simulink model "MMCs_SingleCore"  (R2021b)
settings: Solver=FixedStepDiscrete  StartTime=0.0  StopTime=50  FixedStep=Ts  RelTol=1e-3  EnableMultiTasking=on
InitFcn:
  | MMCs_Parameters;
undefined symbols (not defined in the file): bias, Csm, DiscIntNeverNeededParam, Ki_cc, Ki_E1, Ki_E2, Ki_I, Ki_U, Kp_cc, Kp_E1, Kp_E2, Kp_I, Kp_U, Kr_cc, Kr_I, Kr_U, Nsm, Ts, Vdc, Vout, Vsm, w
libraries: raspberrypiCommlib x7, eeGeneralControl x6, slpidlib x6
settings Model: SimulationMode=external  Creator=s1941852  LastModifiedBy=s1941852
settings SolverCC: PositivePriorityOrder=on  AutoInsertRateTranBlk=on
settings OptimizationCC: EnhancedBackFolding=on  PassReuseOutputArgsAs=Individual arguments  ZeroExternalMemoryAtStartup=off  ZeroInternalMemoryAtStartup=off  MaxStackSize=64  OptimizeBlockOrder=speed  DifferentSizesBufferReuse=on  OptimizationCustomize=off  EfficientTunableParamExpr=on
settings DebuggingCC: ParameterTunabilityLossMsg=error
settings HardwareCC: ProdBitPerPointer=32  ProdBitPerSizeT=32  ProdBitPerPtrDiffT=32  ProdLargestAtomicInteger=Long  ProdLargestAtomicFloat=Double  ProdWordSize=32  ProdLongLongMode=on  ProdHWDeviceType=ARM Compatible->ARM Cortex
settings RTWCC: Description=Embedded Coder  SystemTargetFile=ert.tlc  HardwareBoard=Raspberry Pi  TLCOptions="-aInlineSetEventsForThisBaseRateFcn=TLC_FALSE -aSuppressMultiTaskScheduler=TLC_FALSE  -aRateBasedStepFcn=0"  TemplateMakefile=ert_default_tmf  Toolchain=GNU GCC Embedded Linux  BuildConfiguration=Faster Runs
settings CodeAppCC: ForceParamTrailComments=on  IgnoreCustomStorageClasses=off  OperatorAnnotations=on  SimulinkDataObjDesc=on  SFDataObjDesc=on  InsertBlockDesc=on
settings ERTTargetCC: SupportContinuousTime=on  SupportVariableSizeSignals=on  ExtModeTransport=2  ExtModeStaticAlloc=on  ExtModeMexFile=ext_xcp  ExtModeIntrfLevel=Level2 - Open

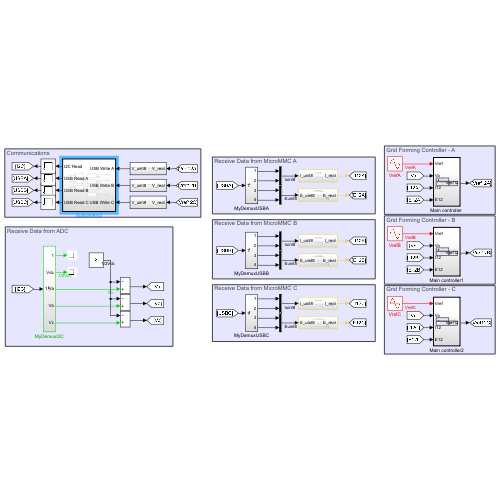
[thumbnail: Simulink's stored preview of the top-level diagram]
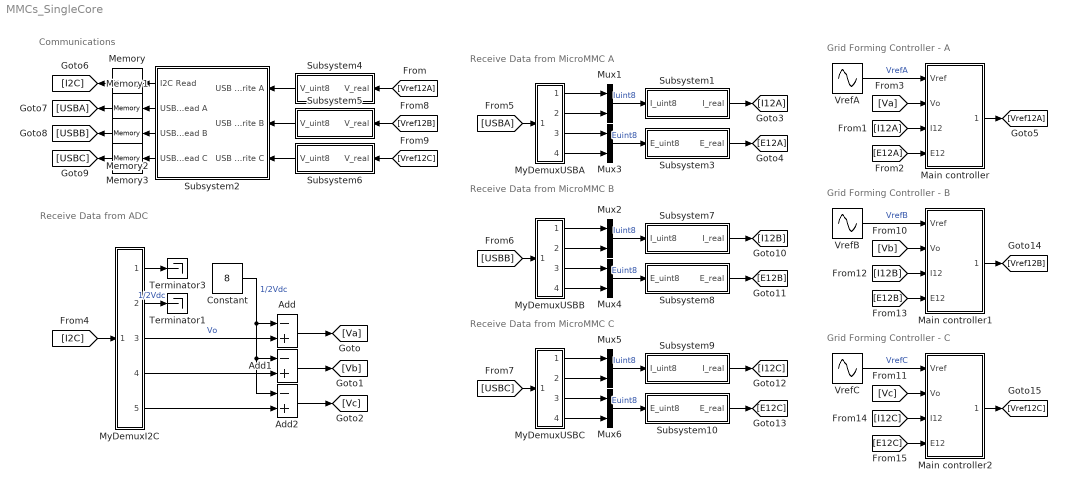
== system MMCs_SingleCore ==
  note: Communications
  note: Grid Forming Controller - A
  note: Receive Data from MicroMMC A
  note: Receive Data from ADC
  note: Grid Forming Controller - B
  note: Grid Forming Controller - C
  note: Receive Data from MicroMMC B
  note: Receive Data from MicroMMC C
  Add : Sum  Inputs=-+
  Add1 : Sum  Inputs=-+
  Add2 : Sum  Inputs=-+
  Constant : Constant  Value=8
  "Main controller " : Subsystem  TreatAsAtomicUnit=on  SystemSampleTime=Ts
  Main controller1 : Subsystem  TreatAsAtomicUnit=on  SystemSampleTime=Ts
  Main controller2 : Subsystem  TreatAsAtomicUnit=on  SystemSampleTime=Ts
  Memory{,1..3} (4 alike) : Memory
  Mux{1..6} (6 alike) : Mux  Inputs=2
  MyDemuxI2C : Subsystem
  MyDemuxUSBA : Subsystem
  MyDemuxUSBB : Subsystem
  MyDemuxUSBC : Subsystem
  Subsystem1 : Subsystem
  Subsystem10 : Subsystem
  Subsystem2 : Subsystem  TreatAsAtomicUnit=on  SystemSampleTime=Ts
      settings: PortSchema="{\"entries\":[{\"content\":{\"sides\":[{\"content\":{\"connectorIds\":[\"Out1\",\"Out2\",\"Out3\",\"Out4\"]},\"type\":\"ConnectorPlacement.EquallySpacedRectSide\",\"uuid\":\"46029ead-0964-4ae9-b883-4a06573532e6\"},{\"content\":{\"connectorIds\":[\"In1\",\"In2\",\"In3\"],\"side\":\"RIGHT\"},\"type\":\"ConnectorPlacement.EquallySpacedRectSide\",\"uuid\":\"15f59cbf-3bfc-4c74-a2e0-6efc08c03cef\"},{\"content\":{\"connectorIds\":[],\"side\":\"TOP\"},\"type\":\"ConnectorPlacement.EquallySpacedRectSide\",\"uuid\":\"8f43b052-da8c-4b5e-b754-50c4f07df149\"}]},\"type\":\"ConnectorPlacement.EquallySpacedConnector\",\"uuid\":\"6541cb38-b92e-4f8c-a13a-509f214bb128\"}],\"packageUris\":[\"http://schema.mathworks.com/mf0/Connector/R2020b\"],\"version\":\"1.0\"}"
  Subsystem3 : Subsystem
  Subsystem4 : Subsystem
  Subsystem5 : Subsystem
  Subsystem6 : Subsystem
  Subsystem7 : Subsystem
  Subsystem8 : Subsystem
  Subsystem9 : Subsystem
  Terminator1 : Terminator
  Terminator3 : Terminator
  VrefA : Sin  Amplitude=Vout  Bias=bias  Frequency=w  SampleTime=0
  VrefB : Sin  Amplitude=Vout  Bias=bias  Frequency=w  Phase=2/3*pi  SampleTime=0
  VrefC : Sin  Amplitude=Vout  Bias=bias  Frequency=w  Phase=4/3*pi  SampleTime=0
  wires:
  MyDemuxUSBA/2(Out2) -> Mux1/2
  MyDemuxUSBA/1(Out1) -> Mux1/1
  Mux1/1 -> Subsystem1/1(I_uint8)  "Iuint8"
  MyDemuxUSBA/4(Out4) -> Mux3/2
  MyDemuxUSBA/3(Out3) -> Mux3/1
  [I2C] -> MyDemuxI2C/1(In1)
  VrefA/1 -> "Main controller "/1(Vref)  "VrefA"
  [USBA] -> MyDemuxUSBA/1(In1)
  MyDemuxI2C/3(Va) -> Add/2  "Vo"
  Subsystem4/1(V_uint8) -> Subsystem2/1(USB Write A)
  MyDemuxI2C/1(Out1) -> Terminator3/1
  MyDemuxI2C/4(Vb) -> Add1/2
  MyDemuxI2C/5(Vc) -> Add2/2
  Mux3/1 -> Subsystem3/1(E_uint8)  "Euint8"
  Constant/1 -> Add/1, Add2/1, Add1/1  "1/2Vdc"
  [Vref12A] -> Subsystem4/1(V_real)
  Add/1 -> [Va]
  Add1/1 -> [Vb]
  Add2/1 -> [Vc]
  Subsystem5/1(V_uint8) -> Subsystem2/2(USB Write B)
  Subsystem6/1(V_uint8) -> Subsystem2/3(USB Write C)
  Subsystem1/1(I_real) -> [I12A]
  Subsystem3/1(E_real) -> [E12A]
  "Main controller "/1(Vref12) -> [Vref12A]
  [I12A] -> "Main controller "/3(I12)
  [E12A] -> "Main controller "/4(E12)
  [Va] -> "Main controller "/2(Vo)
  [Vb] -> Main controller1/2(Vo)
  [E12B] -> Main controller1/4(E12)
  [I12B] -> Main controller1/3(I12)
  Main controller1/1(Vref12) -> [Vref12B]
  VrefB/1 -> Main controller1/1(Vref)  "VrefB"
  VrefC/1 -> Main controller2/1(Vref)  "VrefC"
  Main controller2/1(Vref12) -> [Vref12C]
  [I12C] -> Main controller2/3(I12)
  [E12C] -> Main controller2/4(E12)
  [Vc] -> Main controller2/2(Vo)
  Subsystem8/1(E_real) -> [E12B]
  Subsystem7/1(I_real) -> [I12B]
  Mux4/1 -> Subsystem8/1(E_uint8)  "Euint8"
  MyDemuxUSBB/3(Out3) -> Mux4/1
  MyDemuxUSBB/4(Out4) -> Mux4/2
  Mux2/1 -> Subsystem7/1(I_uint8)  "Iuint8"
  MyDemuxUSBB/1(Out1) -> Mux2/1
  MyDemuxUSBB/2(Out2) -> Mux2/2
  MyDemuxUSBC/2(Out2) -> Mux5/2
  MyDemuxUSBC/1(Out1) -> Mux5/1
  Mux5/1 -> Subsystem9/1(I_uint8)  "Iuint8"
  MyDemuxUSBC/4(Out4) -> Mux6/2
  MyDemuxUSBC/3(Out3) -> Mux6/1
  Mux6/1 -> Subsystem10/1(E_uint8)  "Euint8"
  Subsystem9/1(I_real) -> [I12C]
  Subsystem10/1(E_real) -> [E12C]
  [USBB] -> MyDemuxUSBB/1(In1)
  [USBC] -> MyDemuxUSBC/1(In1)
  [Vref12B] -> Subsystem5/1(V_real)
  [Vref12C] -> Subsystem6/1(V_real)
  MyDemuxI2C/2(Vdc) -> Terminator1/1  "1/2Vdc"
  Memory/1 -> [I2C]
  Subsystem2/1(I2C Read) -> Memory/1
  Memory1/1 -> [USBA]
  Subsystem2/2(USB Read A) -> Memory1/1
  Memory2/1 -> [USBB]
  Subsystem2/3(USB Read B) -> Memory2/1
  Memory3/1 -> [USBC]
  Subsystem2/4(USB Read C) -> Memory3/1

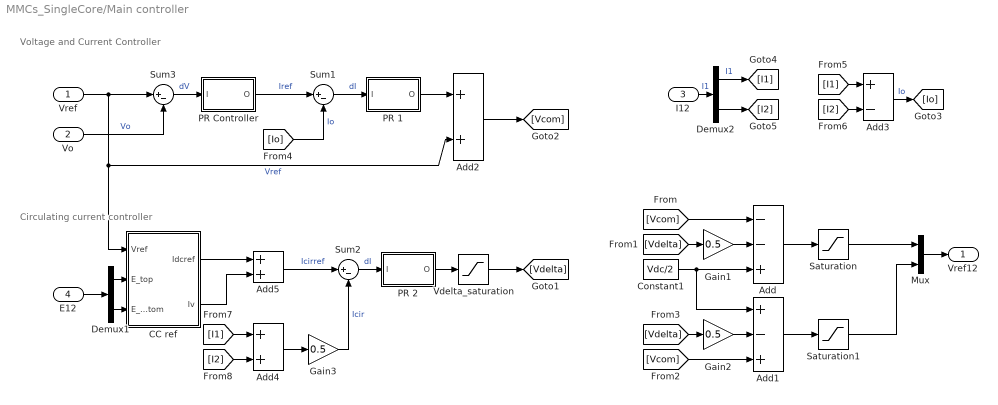
== system MMCs_SingleCore/Main controller  ==
  note: Voltage and Current Controller
  note: Circulating current controller
  Vref : Inport
  Vo : Inport  Port=2
  I12 : Inport  Port=3
  E12 : Inport  Port=4
  Add : Sum  Inputs=--+
  Add1 : Sum  Inputs=+-+
  Add2 : Sum
  Add3 : Sum  Inputs=+-
  Add4 : Sum
  Add5 : Sum
  CC ref : Subsystem
  Constant1 : Constant  Value=Vdc/2
  Demux1 : Demux  Outputs=2
  Demux2 : Demux  Outputs=2
  Gain1 : Gain  Gain=0.5
  Gain2 : Gain  Gain=0.5
  Gain3 : Gain  Gain=0.5
  Mux : Mux  Inputs=2
  PR 1 : Subsystem
  PR 2 : Subsystem
  PR Controller : Subsystem
  Saturation : Saturate  UpperLimit=16  LowerLimit=0
  Saturation1 : Saturate  UpperLimit=16  LowerLimit=0
  Sum1 : Sum  Inputs=|+-
  Sum2 : Sum  Inputs=|+-
  Sum3 : Sum  Inputs=|+-
  Vdelta_saturation : Saturate  UpperLimit=10  LowerLimit=-10
  Vref12 : Outport
  wires:
  Vref/1 -> Sum3/1, Add2/2, CC ref/1(Vref)  "Vref"
  Vo/1 -> Sum3/2  "Vo"
  Sum3/1 -> PR Controller/1(I)  "dV"
  PR Controller/1(O) -> Sum1/1  "Iref"
  [Io] -> Sum1/2  "Io"
  Sum1/1 -> PR 1/1(I)  "dI"
  [Vcom] -> Add/1
  Gain1/1 -> Add/2
  [Vdelta] -> Gain1/1
  [Vcom] -> Add1/3
  [Vdelta] -> Gain2/1
  Gain2/1 -> Add1/2
  Add2/1 -> [Vcom]
  Demux2/2 -> [I2]
  Add3/1 -> [Io]  "Io"
  Sum2/1 -> PR 2/1(I)  "dI"
  [I2] -> Add3/2
  [I1] -> Add3/1
  [I2] -> Add4/2
  Add4/1 -> Gain3/1
  [I1] -> Add4/1
  Add/1 -> Saturation/1
  Add1/1 -> Saturation1/1
  Vdelta_saturation/1 -> [Vdelta]
  Saturation/1 -> Mux/1
  Saturation1/1 -> Mux/2
  Demux2/1 -> [I1]  "I1"
  Constant1/1 -> Add1/1, Add/3
  Demux1/1 -> CC ref/2(E_top)
  Demux1/2 -> CC ref/3(E_bottom)
  Gain3/1 -> Sum2/2  "Icir"
  Add5/1 -> Sum2/1  "Icirref"
  CC ref/1(Idcref) -> Add5/1
  CC ref/2(Iv) -> Add5/2
  PR 1/1(O) -> Add2/1
  PR 2/1(O) -> Vdelta_saturation/1
  E12/1 -> Demux1/1
  I12/1 -> Demux2/1  "I1"
  Mux/1 -> Vref12/1

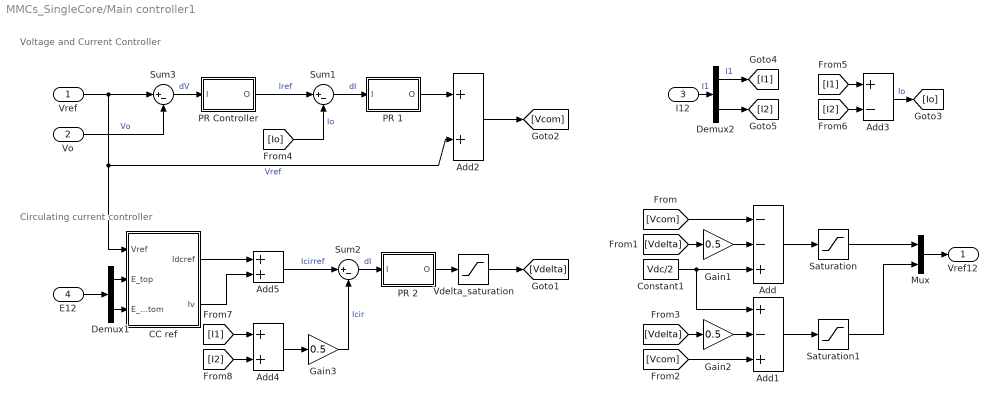
== system MMCs_SingleCore/Main controller1 ==
  note: Circulating current controller
  note: Voltage and Current Controller
  Vref : Inport
  Vo : Inport  Port=2
  I12 : Inport  Port=3
  E12 : Inport  Port=4
  Add : Sum  Inputs=--+
  Add1 : Sum  Inputs=+-+
  Add2 : Sum
  Add3 : Sum  Inputs=+-
  Add4 : Sum
  Add5 : Sum
  CC ref : Subsystem
  Constant1 : Constant  Value=Vdc/2
  Demux1 : Demux  Outputs=2
  Demux2 : Demux  Outputs=2
  Gain1 : Gain  Gain=0.5
  Gain2 : Gain  Gain=0.5
  Gain3 : Gain  Gain=0.5
  Mux : Mux  Inputs=2
  PR 1 : Subsystem
  PR 2 : Subsystem
  PR Controller : Subsystem
  Saturation : Saturate  UpperLimit=16  LowerLimit=0
  Saturation1 : Saturate  UpperLimit=16  LowerLimit=0
  Sum1 : Sum  Inputs=|+-
  Sum2 : Sum  Inputs=|+-
  Sum3 : Sum  Inputs=|+-
  Vdelta_saturation : Saturate  UpperLimit=10  LowerLimit=-10
  Vref12 : Outport
  wires:
  Mux/1 -> Vref12/1
  I12/1 -> Demux2/1  "I1"
  E12/1 -> Demux1/1
  PR 2/1(O) -> Vdelta_saturation/1
  PR 1/1(O) -> Add2/1
  CC ref/2(Iv) -> Add5/2
  CC ref/1(Idcref) -> Add5/1
  Add5/1 -> Sum2/1  "Icirref"
  Gain3/1 -> Sum2/2  "Icir"
  Demux1/2 -> CC ref/3(E_bottom)
  Demux1/1 -> CC ref/2(E_top)
  Constant1/1 -> Add/3, Add1/1
  Demux2/1 -> [I1]  "I1"
  Saturation1/1 -> Mux/2
  Saturation/1 -> Mux/1
  Vdelta_saturation/1 -> [Vdelta]
  Add1/1 -> Saturation1/1
  Add/1 -> Saturation/1
  [I1] -> Add4/1
  Add4/1 -> Gain3/1
  [I2] -> Add4/2
  [I1] -> Add3/1
  [I2] -> Add3/2
  Sum2/1 -> PR 2/1(I)  "dI"
  Add3/1 -> [Io]  "Io"
  Demux2/2 -> [I2]
  Add2/1 -> [Vcom]
  Gain2/1 -> Add1/2
  [Vdelta] -> Gain2/1
  [Vcom] -> Add1/3
  [Vdelta] -> Gain1/1
  Gain1/1 -> Add/2
  [Vcom] -> Add/1
  Sum1/1 -> PR 1/1(I)  "dI"
  [Io] -> Sum1/2  "Io"
  PR Controller/1(O) -> Sum1/1  "Iref"
  Sum3/1 -> PR Controller/1(I)  "dV"
  Vo/1 -> Sum3/2  "Vo"
  Vref/1 -> CC ref/1(Vref), Add2/2, Sum3/1  "Vref"

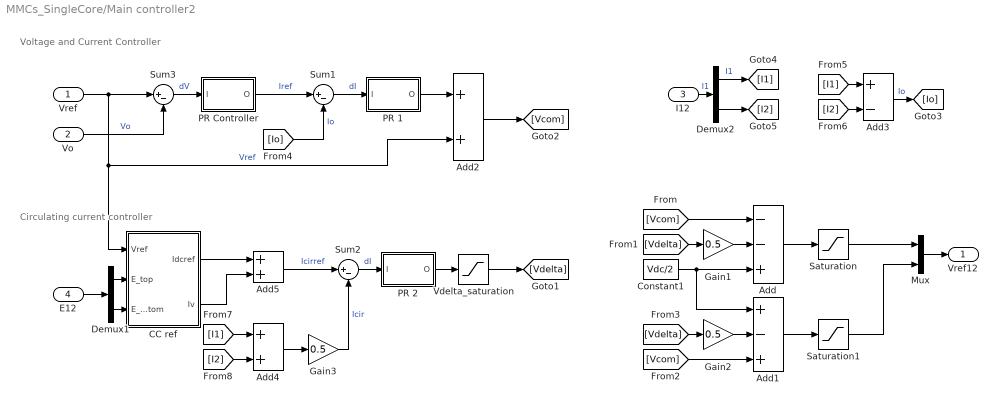
== system MMCs_SingleCore/Main controller2 ==
  note: Voltage and Current Controller
  note: Circulating current controller
  Vref : Inport
  Vo : Inport  Port=2
  I12 : Inport  Port=3
  E12 : Inport  Port=4
  Add : Sum  Inputs=--+
  Add1 : Sum  Inputs=+-+
  Add2 : Sum
  Add3 : Sum  Inputs=+-
  Add4 : Sum
  Add5 : Sum
  CC ref : Subsystem
  Constant1 : Constant  Value=Vdc/2
  Demux1 : Demux  Outputs=2
  Demux2 : Demux  Outputs=2
  Gain1 : Gain  Gain=0.5
  Gain2 : Gain  Gain=0.5
  Gain3 : Gain  Gain=0.5
  Mux : Mux  Inputs=2
  PR 1 : Subsystem
  PR 2 : Subsystem
  PR Controller : Subsystem
  Saturation : Saturate  UpperLimit=16  LowerLimit=0
  Saturation1 : Saturate  UpperLimit=16  LowerLimit=0
  Sum1 : Sum  Inputs=|+-
  Sum2 : Sum  Inputs=|+-
  Sum3 : Sum  Inputs=|+-
  Vdelta_saturation : Saturate  UpperLimit=10  LowerLimit=-10
  Vref12 : Outport
  wires:
  Vref/1 -> Sum3/1, Add2/2, CC ref/1(Vref)  "Vref"
  Vo/1 -> Sum3/2  "Vo"
  Sum3/1 -> PR Controller/1(I)  "dV"
  PR Controller/1(O) -> Sum1/1  "Iref"
  [Io] -> Sum1/2  "Io"
  Sum1/1 -> PR 1/1(I)  "dI"
  [Vcom] -> Add/1
  Gain1/1 -> Add/2
  [Vdelta] -> Gain1/1
  [Vcom] -> Add1/3
  [Vdelta] -> Gain2/1
  Gain2/1 -> Add1/2
  Add2/1 -> [Vcom]
  Demux2/2 -> [I2]
  Add3/1 -> [Io]  "Io"
  Sum2/1 -> PR 2/1(I)  "dI"
  [I2] -> Add3/2
  [I1] -> Add3/1
  [I2] -> Add4/2
  Add4/1 -> Gain3/1
  [I1] -> Add4/1
  Add/1 -> Saturation/1
  Add1/1 -> Saturation1/1
  Vdelta_saturation/1 -> [Vdelta]
  Saturation/1 -> Mux/1
  Saturation1/1 -> Mux/2
  Demux2/1 -> [I1]  "I1"
  Constant1/1 -> Add1/1, Add/3
  Demux1/1 -> CC ref/2(E_top)
  Demux1/2 -> CC ref/3(E_bottom)
  Gain3/1 -> Sum2/2  "Icir"
  Add5/1 -> Sum2/1  "Icirref"
  CC ref/1(Idcref) -> Add5/1
  CC ref/2(Iv) -> Add5/2
  PR 1/1(O) -> Add2/1
  PR 2/1(O) -> Vdelta_saturation/1
  E12/1 -> Demux1/1
  I12/1 -> Demux2/1  "I1"
  Mux/1 -> Vref12/1

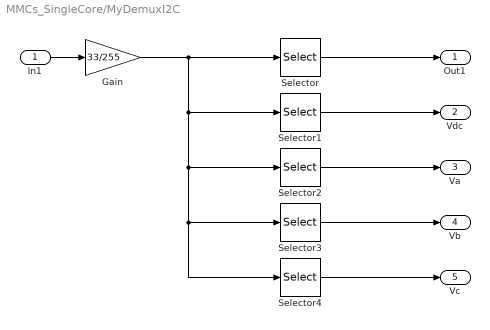
== system MMCs_SingleCore/MyDemuxI2C ==
  In1 : Inport
  Gain : Gain  Gain=33/255
  Selector : Selector  NumberOfDimensions=2  InputPortWidth=4  IndexOptions=Index vector (dialog),Index vector (dialog)  Indices=[1],1  OutputSizes=1,1
  Selector1 : Selector  NumberOfDimensions=2  InputPortWidth=4  IndexOptions=Index vector (dialog),Index vector (dialog)  Indices=[2],1  OutputSizes=1,1
  Selector2 : Selector  NumberOfDimensions=2  InputPortWidth=4  IndexOptions=Index vector (dialog),Index vector (dialog)  Indices=[3],1  OutputSizes=1,1
  Selector3 : Selector  NumberOfDimensions=2  InputPortWidth=4  IndexOptions=Index vector (dialog),Index vector (dialog)  Indices=[4],1  OutputSizes=1,1
  Selector4 : Selector  NumberOfDimensions=2  InputPortWidth=4  IndexOptions=Index vector (dialog),Index vector (dialog)  Indices=[5],1  OutputSizes=1,1
  Out1 : Outport
  Vdc : Outport  Port=2
  Va : Outport  Port=3
  Vb : Outport  Port=4
  Vc : Outport  Port=5
  wires:
  In1/1 -> Gain/1
  Selector1/1 -> Vdc/1
  Selector2/1 -> Va/1
  Selector3/1 -> Vb/1
  Selector/1 -> Out1/1
  Selector4/1 -> Vc/1
  Gain/1 -> Selector4/1, Selector3/1, Selector2/1, Selector1/1, Selector/1

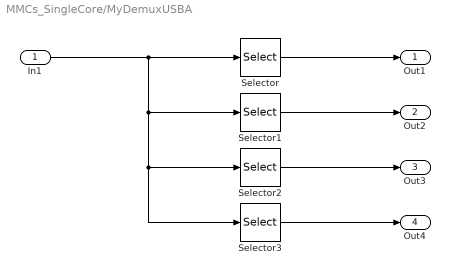
== system MMCs_SingleCore/MyDemuxUSBA ==
  In1 : Inport
  Selector : Selector  NumberOfDimensions=2  InputPortWidth=4  IndexOptions=Index vector (dialog),Index vector (dialog)  Indices=[1],1  OutputSizes=1,1
  Selector1 : Selector  NumberOfDimensions=2  InputPortWidth=4  IndexOptions=Index vector (dialog),Index vector (dialog)  Indices=[2],1  OutputSizes=1,1
  Selector2 : Selector  NumberOfDimensions=2  InputPortWidth=4  IndexOptions=Index vector (dialog),Index vector (dialog)  Indices=[3],1  OutputSizes=1,1
  Selector3 : Selector  NumberOfDimensions=2  InputPortWidth=4  IndexOptions=Index vector (dialog),Index vector (dialog)  Indices=[4],1  OutputSizes=1,1
  Out1 : Outport
  Out2 : Outport  Port=2
  Out3 : Outport  Port=3
  Out4 : Outport  Port=4
  wires:
  In1/1 -> Selector3/1, Selector2/1, Selector1/1, Selector/1
  Selector1/1 -> Out2/1
  Selector2/1 -> Out3/1
  Selector3/1 -> Out4/1
  Selector/1 -> Out1/1

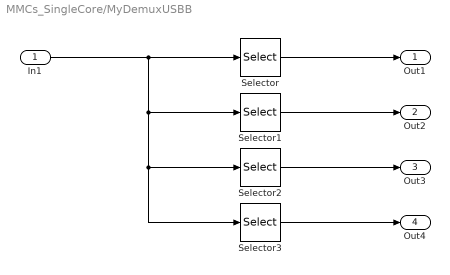
== system MMCs_SingleCore/MyDemuxUSBB ==
  In1 : Inport
  Selector : Selector  NumberOfDimensions=2  InputPortWidth=4  IndexOptions=Index vector (dialog),Index vector (dialog)  Indices=[1],1  OutputSizes=1,1
  Selector1 : Selector  NumberOfDimensions=2  InputPortWidth=4  IndexOptions=Index vector (dialog),Index vector (dialog)  Indices=[2],1  OutputSizes=1,1
  Selector2 : Selector  NumberOfDimensions=2  InputPortWidth=4  IndexOptions=Index vector (dialog),Index vector (dialog)  Indices=[3],1  OutputSizes=1,1
  Selector3 : Selector  NumberOfDimensions=2  InputPortWidth=4  IndexOptions=Index vector (dialog),Index vector (dialog)  Indices=[4],1  OutputSizes=1,1
  Out1 : Outport
  Out2 : Outport  Port=2
  Out3 : Outport  Port=3
  Out4 : Outport  Port=4
  wires:
  Selector/1 -> Out1/1
  Selector3/1 -> Out4/1
  Selector2/1 -> Out3/1
  Selector1/1 -> Out2/1
  In1/1 -> Selector/1, Selector1/1, Selector2/1, Selector3/1

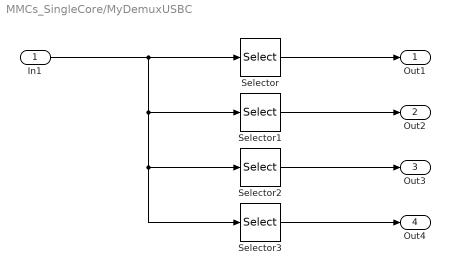
== system MMCs_SingleCore/MyDemuxUSBC ==
  In1 : Inport
  Selector : Selector  NumberOfDimensions=2  InputPortWidth=4  IndexOptions=Index vector (dialog),Index vector (dialog)  Indices=[1],1  OutputSizes=1,1
  Selector1 : Selector  NumberOfDimensions=2  InputPortWidth=4  IndexOptions=Index vector (dialog),Index vector (dialog)  Indices=[2],1  OutputSizes=1,1
  Selector2 : Selector  NumberOfDimensions=2  InputPortWidth=4  IndexOptions=Index vector (dialog),Index vector (dialog)  Indices=[3],1  OutputSizes=1,1
  Selector3 : Selector  NumberOfDimensions=2  InputPortWidth=4  IndexOptions=Index vector (dialog),Index vector (dialog)  Indices=[4],1  OutputSizes=1,1
  Out1 : Outport
  Out2 : Outport  Port=2
  Out3 : Outport  Port=3
  Out4 : Outport  Port=4
  wires:
  In1/1 -> Selector3/1, Selector2/1, Selector1/1, Selector/1
  Selector1/1 -> Out2/1
  Selector2/1 -> Out3/1
  Selector3/1 -> Out4/1
  Selector/1 -> Out1/1

== system MMCs_SingleCore/Subsystem1 ==
  note: (-3 to 3) --> (0 to 240)
      | (I_real + 3) * 40 = I_uint8
  I_uint8 : Inport
  Constant : Constant  Value=3  SampleTime=-1
  Convert to double : DataTypeConversion  OutDataTypeStr=double
  Gain : Gain  Gain=1/40
  Sum3 : Sum  Inputs=+-
  I_real : Outport
  wires:
  Gain/1 -> Sum3/1
  Convert to double/1 -> Gain/1
  Constant/1 -> Sum3/2
  I_uint8/1 -> Convert to double/1
  Sum3/1 -> I_real/1

== system MMCs_SingleCore/Subsystem10 ==
  note: (0 to 2.4) --> (0 to 120)
      | E_real * 50 = E_uint8
      | 4 * 1/2 * 3 * 6.8e-3 * 5^2 = 1.02 (51 in uint8)
  E_uint8 : Inport
  Convert to double : DataTypeConversion  OutDataTypeStr=double
  Gain : Gain  Gain=1/50
  Scope : Scope  NumInputPorts=3
  E_real : Outport
  wires:
  Gain/1 -> Scope/3, E_real/1
  E_uint8/1 -> Scope/1, Convert to double/1
  Convert to double/1 -> Scope/2, Gain/1

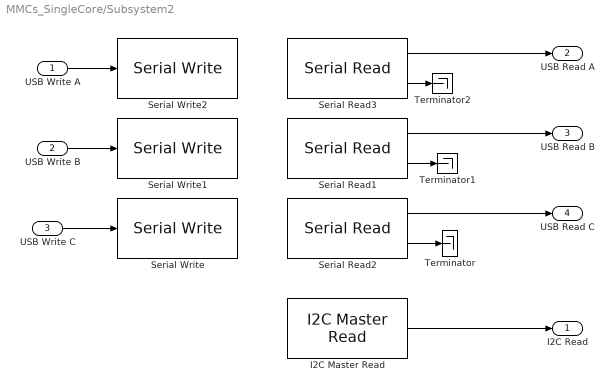
== system MMCs_SingleCore/Subsystem2 ==
  USB Write A : Inport
  USB Write B : Inport  Port=2
  USB Write C : Inport  Port=3
  I2C Master Read : raspberrypiCommlib/I2C Master Read  Priority=1  BoardProperty=Pi 4 Model B  Mode=Master  SlaveAddress=hex2dec('20')  SlaveByteOrder=BigEndian  Direction=Receiver  RegisterAddressMode=off  RegisterAddress=0b00000000  SlaveDataType=uint8  DataLength=5  NoAck=off  RepeatedStart=off  OutputStatus=off  SampleTime=-1
      settings: SourceProductBaseCode=RASPPI
  Serial Read1 : raspberrypiCommlib/Serial Read  Priority=5  board=Pi 4 Model B  SCIModule_=/dev/ttyACM1  Baudrate_=230400  Parity=None  StopBits_=1  HardwareFlowControl=None  ByteOrder=LittleEndian  DataLength=4  DataType=uint8  OutputStatus=on  SampleTime=-1  blockPlatform=RaspberryPi
      settings: SourceProductBaseCode=RASPPI
  Serial Read2 : raspberrypiCommlib/Serial Read  Priority=7  board=Pi 4 Model B  SCIModule_=/dev/ttyACM2  Baudrate_=230400  Parity=None  StopBits_=1  HardwareFlowControl=None  ByteOrder=LittleEndian  DataLength=4  DataType=uint8  OutputStatus=on  SampleTime=-1  blockPlatform=RaspberryPi
      settings: SourceProductBaseCode=RASPPI
  Serial Read3 : raspberrypiCommlib/Serial Read  Priority=3  board=Pi 4 Model B  SCIModule_=/dev/ttyACM0  Baudrate_=230400  Parity=None  StopBits_=1  HardwareFlowControl=None  ByteOrder=LittleEndian  DataLength=4  DataType=uint8  OutputStatus=on  SampleTime=-1  blockPlatform=RaspberryPi
      settings: SourceProductBaseCode=RASPPI
  Serial Write : raspberrypiCommlib/Serial Write  Priority=6  board=Pi 4 Model B  SCIModule_=/dev/ttyACM2  Baudrate_=230400  Parity=None  StopBits_=1  HardwareFlowControl=None  ByteOrder=LittleEndian  OutputStatus=off  blockPlatform=RaspberryPi
      settings: SourceProductBaseCode=RASPPI
  Serial Write1 : raspberrypiCommlib/Serial Write  Priority=4  board=Pi 4 Model B  SCIModule_=/dev/ttyACM1  Baudrate_=230400  Parity=None  StopBits_=1  HardwareFlowControl=None  ByteOrder=LittleEndian  OutputStatus=off  blockPlatform=RaspberryPi
      settings: SourceProductBaseCode=RASPPI
  Serial Write2 : raspberrypiCommlib/Serial Write  Priority=2  board=Pi 4 Model B  SCIModule_=/dev/ttyACM0  Baudrate_=230400  Parity=None  StopBits_=1  HardwareFlowControl=None  ByteOrder=LittleEndian  OutputStatus=off  blockPlatform=RaspberryPi
      settings: SourceProductBaseCode=RASPPI
  Terminator : Terminator
  Terminator1 : Terminator
  Terminator2 : Terminator
  I2C Read : Outport
  USB Read A : Outport  Port=2
  USB Read B : Outport  Port=3
  USB Read C : Outport  Port=4
  wires:
  I2C Master Read/1 -> I2C Read/1
  Serial Read2/2 -> Terminator/1
  Serial Read1/2 -> Terminator1/1
  Serial Read3/2 -> Terminator2/1
  USB Write A/1 -> Serial Write2/1
  Serial Read2/1 -> USB Read C/1
  USB Write B/1 -> Serial Write1/1
  Serial Read1/1 -> USB Read B/1
  USB Write C/1 -> Serial Write/1
  Serial Read3/1 -> USB Read A/1

== system MMCs_SingleCore/Subsystem3 ==
  note: (0 to 2.4) --> (0 to 120)
      | E_real * 50 = E_uint8
      | 4 * 1/2 * 3 * 6.8e-3 * 5^2 = 1.02 (51 in uint8)
  E_uint8 : Inport
  Convert to double : DataTypeConversion  OutDataTypeStr=double
  Gain : Gain  Gain=1/50
  Scope : Scope  NumInputPorts=3
  E_real : Outport
  wires:
  Gain/1 -> Scope/3, E_real/1
  E_uint8/1 -> Scope/1, Convert to double/1
  Convert to double/1 -> Scope/2, Gain/1

== system MMCs_SingleCore/Subsystem4 ==
  V_real : Inport
  Add : Sum
  Constant3 : Constant  Value=20
  Convert to logical1 : DataTypeConversion  OutDataTypeStr=uint8
  Gain : Gain  Gain=240/40
  Saturation1 : Saturate  UpperLimit=2^8-1  LowerLimit=0
  V_uint8 : Outport
  wires:
  Constant3/1 -> Add/2
  Convert to logical1/1 -> V_uint8/1
  Saturation1/1 -> Convert to logical1/1
  V_real/1 -> Add/1
  Add/1 -> Gain/1
  Gain/1 -> Saturation1/1

== system MMCs_SingleCore/Subsystem5 ==
  V_real : Inport
  Add : Sum
  Constant3 : Constant  Value=20
  Convert to logical1 : DataTypeConversion  OutDataTypeStr=uint8
  Gain : Gain  Gain=240/40
  Saturation1 : Saturate  UpperLimit=2^8-1  LowerLimit=0
  V_uint8 : Outport
  wires:
  Gain/1 -> Saturation1/1
  Add/1 -> Gain/1
  V_real/1 -> Add/1
  Saturation1/1 -> Convert to logical1/1
  Convert to logical1/1 -> V_uint8/1
  Constant3/1 -> Add/2

== system MMCs_SingleCore/Subsystem6 ==
  V_real : Inport
  Add : Sum
  Constant3 : Constant  Value=20
  Convert to logical1 : DataTypeConversion  OutDataTypeStr=uint8
  Gain : Gain  Gain=240/40
  Saturation1 : Saturate  UpperLimit=2^8-1  LowerLimit=0
  V_uint8 : Outport
  wires:
  Constant3/1 -> Add/2
  Convert to logical1/1 -> V_uint8/1
  Saturation1/1 -> Convert to logical1/1
  V_real/1 -> Add/1
  Add/1 -> Gain/1
  Gain/1 -> Saturation1/1

== system MMCs_SingleCore/Subsystem7 ==
  note: (-3 to 3) --> (0 to 240)
      | (I_real + 3) * 40 = I_uint8
  I_uint8 : Inport
  Constant : Constant  Value=3  SampleTime=-1
  Convert to double : DataTypeConversion  OutDataTypeStr=double
  Gain : Gain  Gain=1/40
  Sum3 : Sum  Inputs=+-
  I_real : Outport
  wires:
  Sum3/1 -> I_real/1
  I_uint8/1 -> Convert to double/1
  Constant/1 -> Sum3/2
  Convert to double/1 -> Gain/1
  Gain/1 -> Sum3/1

== system MMCs_SingleCore/Subsystem8 ==
  note: (0 to 2.4) --> (0 to 120)
      | E_real * 50 = E_uint8
      | 4 * 1/2 * 3 * 6.8e-3 * 5^2 = 1.02 (51 in uint8)
  E_uint8 : Inport
  Convert to double : DataTypeConversion  OutDataTypeStr=double
  Gain : Gain  Gain=1/50
  Scope : Scope  NumInputPorts=3
  E_real : Outport
  wires:
  Convert to double/1 -> Gain/1, Scope/2
  E_uint8/1 -> Convert to double/1, Scope/1
  Gain/1 -> E_real/1, Scope/3

== system MMCs_SingleCore/Subsystem9 ==
  note: (-3 to 3) --> (0 to 240)
      | (I_real + 3) * 40 = I_uint8
  I_uint8 : Inport
  Constant : Constant  Value=3  SampleTime=-1
  Convert to double : DataTypeConversion  OutDataTypeStr=double
  Gain : Gain  Gain=1/40
  Sum3 : Sum  Inputs=+-
  I_real : Outport
  wires:
  Gain/1 -> Sum3/1
  Convert to double/1 -> Gain/1
  Constant/1 -> Sum3/2
  I_uint8/1 -> Convert to double/1
  Sum3/1 -> I_real/1

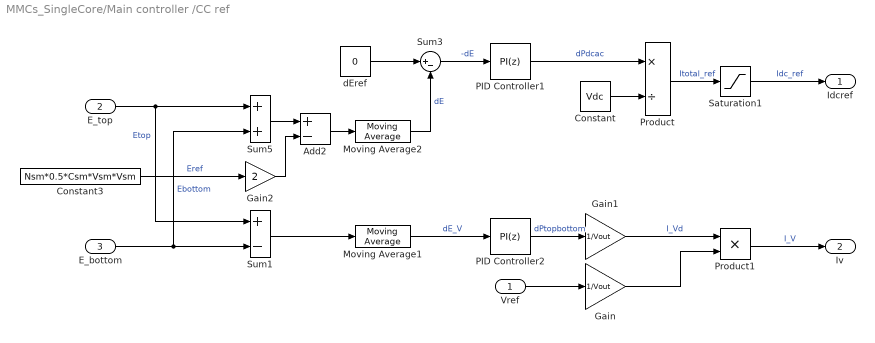
== system MMCs_SingleCore/Main controller /CC ref ==
  Vref : Inport
  E_top : Inport  Port=2
  E_bottom : Inport  Port=3
  Add2 : Sum  Inputs=+-
  Constant : Constant  Value=Vdc
  Constant3 : Constant  Value=Nsm*0.5*Csm*Vsm*Vsm
  Gain : Gain  Gain=1/Vout
  Gain1 : Gain  Gain=1/Vout
  Gain2 : Gain  Gain=2
  Moving Average1 : eeGeneralControl/Moving Average  VariantControl=Variant1  LabelModeActiveChoice=Discrete  f=5  x0=0  BufferSize=8192  Ts=Ts
      settings: SourceProductBaseCode=PS
  Moving Average2 : eeGeneralControl/Moving Average  VariantControl=Variant1  LabelModeActiveChoice=Discrete  f=5  x0=0  BufferSize=8192  Ts=Ts
      settings: SourceProductBaseCode=PS
  PID Controller1 : slpidlib/PID Controller  Controller=PI  Form=Parallel  TimeDomain=Discrete-time  UseExternalTs=off  SampleTime=-1  IntegratorMethod=Forward Euler  FilterMethod=Forward Euler  ControllerParametersSource=internal  P=Kp_E1  I=Ki_E1  D=0  UseFilter=on  N=100  TunerSelectOption=Transfer Function Based (PID Tuner App)  InitialConditionSource=internal  InitialConditionForIntegrator=0  InitialConditionForFilter=0  DifferentiatorICPrevScaledInput=0  ExternalReset=none  TrackingMode=off  Kt=1  LimitOutput=off  SatLimitsSource=internal  UpperSaturationLimit=inf  LowerSaturationLimit=-inf  LinearizeAsGain=on  AntiWindupMode=none  Kb=1  POutMin=[]  POutMax=[]  IOutMin=[]  IOutMax=[]  DOutMin=[]  DOutMax=[]  NOutMin=[]  NOutMax=[]  SumOutMin=[]  SumOutMax=[]  SaturationOutMin=[]  SaturationOutMax=[]  PParamMin=[]  PParamMax=[]  IParamMin=[]  IParamMax=[]  DParamMin=[]  DParamMax=[]  NParamMin=[]  NParamMax=[]  KbParamMin=[]  KbParamMax=[]  KtParamMin=[]  KtParamMax=[]  KbOutMin=[]  KbOutMax=[]  KtOutMin=[]  KtOutMax=[]  IntegratorOutMin=[]  IntegratorOutMax=[]  FilterOutMin=[]  FilterOutMax=[]  SumI1OutMin=[]  SumI1OutMax=[]  SumI2OutMin=[]  SumI2OutMax=[]  SumI3OutMin=[]  SumI3OutMax=[]  SumI4OutMin=[]  SumI4OutMax=[]  SumDOutMin=[]  SumDOutMax=[]  DifferentiatorOutMin=[]  DifferentiatorOutMax=[]  FilterDiffOutCoefMin=[]  FilterDiffOutCoefMax=[]  ReciprocalOutMin=[]  ReciprocalOutMax=[]  SumDenOutMin=[]  SumDenOutMax=[]  SumNumOutMin=[]  SumNumOutMax=[]  DivideOutMin=[]  DivideOutMax=[]  UdiffTsProdOutMin=[]  UdiffTsProdOutMax=[]  NTsProdOutMin=[]  NTsProdOutMax=[]  UintegralTsProdOutMin=[]  UintegralTsProdOutMax=[]  UngainTsProdOutMin=[]  UngainTsProdOutMax=[]  IntegratorContinuousStateAttributes=''  IntegratorStateMustResolveToSignalObject=off  IntegratorRTWStateStorageClass=Auto  FilterContinuousStateAttributes=''  FilterStateMustResolveToSignalObject=off  FilterRTWStateStorageClass=Auto  ParallelPVariant=InternalParameters  IdealPVariant=Disabled  IVariant=InternalParameters  DVariant=Disabled  IntegratorVariant=Discrete  SatVariant=Disabled  AWVariant=Passthrough  PCopyVariant=Disabled  TRVariant=Disabled  FdbkBlocksVariant=Forward  IdealPFdbkVariant=Disabled  SatFdbkVariant=Disabled  DerivativeFilterVariant=Disabled  NVariant=Disabled  NCopyVariant=Disabled_SignalSpec  FilterICVariant=Disabled  IntegratorICVariant=InternalICs  ExternalResetVariant=Disabled  TRSumVariant=Passthrough  SumFdbkVariant=Disabled  SumVariant=Sum_PI  TsampFilterVariant=InternalTs  TsampNgainVariant=Passthrough  TsampIntegralVariant=Passthrough  ExternalSaturationOutDataTypeStr=Inherit: Same as second input
  PID Controller2 : slpidlib/PID Controller  Controller=PI  Form=Parallel  TimeDomain=Discrete-time  UseExternalTs=off  SampleTime=-1  IntegratorMethod=Forward Euler  FilterMethod=Forward Euler  ControllerParametersSource=internal  P=Kp_E2  I=Ki_E2  D=0  UseFilter=on  N=100  TunerSelectOption=Transfer Function Based (PID Tuner App)  InitialConditionSource=internal  InitialConditionForIntegrator=0  InitialConditionForFilter=0  DifferentiatorICPrevScaledInput=0  ExternalReset=none  TrackingMode=off  Kt=1  LimitOutput=off  SatLimitsSource=internal  UpperSaturationLimit=inf  LowerSaturationLimit=-inf  LinearizeAsGain=on  AntiWindupMode=none  Kb=1  POutMin=[]  POutMax=[]  IOutMin=[]  IOutMax=[]  DOutMin=[]  DOutMax=[]  NOutMin=[]  NOutMax=[]  SumOutMin=[]  SumOutMax=[]  SaturationOutMin=[]  SaturationOutMax=[]  PParamMin=[]  PParamMax=[]  IParamMin=[]  IParamMax=[]  DParamMin=[]  DParamMax=[]  NParamMin=[]  NParamMax=[]  KbParamMin=[]  KbParamMax=[]  KtParamMin=[]  KtParamMax=[]  KbOutMin=[]  KbOutMax=[]  KtOutMin=[]  KtOutMax=[]  IntegratorOutMin=[]  IntegratorOutMax=[]  FilterOutMin=[]  FilterOutMax=[]  SumI1OutMin=[]  SumI1OutMax=[]  SumI2OutMin=[]  SumI2OutMax=[]  SumI3OutMin=[]  SumI3OutMax=[]  SumI4OutMin=[]  SumI4OutMax=[]  SumDOutMin=[]  SumDOutMax=[]  DifferentiatorOutMin=[]  DifferentiatorOutMax=[]  FilterDiffOutCoefMin=[]  FilterDiffOutCoefMax=[]  ReciprocalOutMin=[]  ReciprocalOutMax=[]  SumDenOutMin=[]  SumDenOutMax=[]  SumNumOutMin=[]  SumNumOutMax=[]  DivideOutMin=[]  DivideOutMax=[]  UdiffTsProdOutMin=[]  UdiffTsProdOutMax=[]  NTsProdOutMin=[]  NTsProdOutMax=[]  UintegralTsProdOutMin=[]  UintegralTsProdOutMax=[]  UngainTsProdOutMin=[]  UngainTsProdOutMax=[]  IntegratorContinuousStateAttributes=''  IntegratorStateMustResolveToSignalObject=off  IntegratorRTWStateStorageClass=Auto  FilterContinuousStateAttributes=''  FilterStateMustResolveToSignalObject=off  FilterRTWStateStorageClass=Auto  ParallelPVariant=InternalParameters  IdealPVariant=Disabled  IVariant=InternalParameters  DVariant=Disabled  IntegratorVariant=Discrete  SatVariant=Disabled  AWVariant=Passthrough  PCopyVariant=Disabled  TRVariant=Disabled  FdbkBlocksVariant=Forward  IdealPFdbkVariant=Disabled  SatFdbkVariant=Disabled  DerivativeFilterVariant=Disabled  NVariant=Disabled  NCopyVariant=Disabled_SignalSpec  FilterICVariant=Disabled  IntegratorICVariant=InternalICs  ExternalResetVariant=Disabled  TRSumVariant=Passthrough  SumFdbkVariant=Disabled  SumVariant=Sum_PI  TsampFilterVariant=InternalTs  TsampNgainVariant=Passthrough  TsampIntegralVariant=Passthrough  ExternalSaturationOutDataTypeStr=Inherit: Same as second input
  Product : Product  Inputs=*/  InputSameDT=on  SaturateOnIntegerOverflow=on  OutDataTypeStr=Inherit: Same as first input
  Product1 : Product
  Saturation1 : Saturate  UpperLimit=1  LowerLimit=-1
  Sum1 : Sum  Inputs=+-
  Sum3 : Sum  Inputs=|+-
  Sum5 : Sum
  dEref : Constant  Value=0
  Idcref : Outport
  Iv : Outport  Port=2
  wires:
  Vref/1 -> Gain/1
  Constant/1 -> Product/2
  Sum5/1 -> Add2/1
  Moving Average2/1 -> Sum3/2  "dE"
  dEref/1 -> Sum3/1
  Sum3/1 -> PID Controller1/1  "-dE"
  PID Controller1/1 -> Product/1  "dPdcac"
  Sum1/1 -> Moving Average1/1
  Moving Average1/1 -> PID Controller2/1  "dE_V"
  PID Controller2/1 -> Gain1/1  "dPtopbottom"
  Saturation1/1 -> Idcref/1  "Idc_ref"
  E_top/1 -> Sum5/1, Sum1/1  "Etop"
  E_bottom/1 -> Sum5/2, Sum1/2  "Ebottom"
  Product1/1 -> Iv/1  "I_V"
  Gain/1 -> Product1/2
  Product/1 -> Saturation1/1  "Itotal_ref"
  Gain1/1 -> Product1/1  "I_Vd"
  Constant3/1 -> Gain2/1  "Eref"
  Gain2/1 -> Add2/2
  Add2/1 -> Moving Average2/1

== system MMCs_SingleCore/Main controller /PR 1 ==
  I : Inport
  Add : Sum  Inputs=+++
  Discrete Transfer Fcn : DiscreteTransferFcn  Numerator=[1 -cos(w*Ts) 0]  Denominator=[1 -2*cos(w*Ts) 1]
  Discrete-Time Integrator : DiscreteIntegrator  gainval=1  SampleTime=-1  ICPrevOutput=DiscIntNeverNeededParam  ICPrevScaledInput=DiscIntNeverNeededParam
  Gain1 : Gain  Gain=Kp_I
  Gain2 : Gain  Gain=Kr_I
  Gain3 : Gain  Gain=Ki_I
  O : Outport
  wires:
  Add/1 -> O/1
  I/1 -> Gain2/1, Gain3/1, Gain1/1
  Gain1/1 -> Add/1
  Gain2/1 -> Discrete Transfer Fcn/1
  Discrete Transfer Fcn/1 -> Add/3
  Gain3/1 -> Discrete-Time Integrator/1
  Discrete-Time Integrator/1 -> Add/2

== system MMCs_SingleCore/Main controller /PR 2 ==
  I : Inport
  Add : Sum  Inputs=+++
  Discrete Transfer Fcn : DiscreteTransferFcn  Numerator=[1 -cos(w*Ts) 0]  Denominator=[1 -2*cos(w*Ts) 1]
  Discrete-Time Integrator : DiscreteIntegrator  gainval=1  SampleTime=-1  ICPrevOutput=DiscIntNeverNeededParam  ICPrevScaledInput=DiscIntNeverNeededParam
  Gain1 : Gain  Gain=Kp_cc
  Gain2 : Gain  Gain=Kr_cc
  Gain3 : Gain  Gain=Ki_cc
  O : Outport
  wires:
  Gain2/1 -> Discrete Transfer Fcn/1
  Gain1/1 -> Add/1  "P"
  I/1 -> Gain2/1, Gain3/1, Gain1/1  "In"
  Discrete Transfer Fcn/1 -> Add/3  "R"
  Add/1 -> O/1
  Gain3/1 -> Discrete-Time Integrator/1
  Discrete-Time Integrator/1 -> Add/2  "I"

== system MMCs_SingleCore/Main controller /PR Controller ==
  I : Inport
  Add : Sum  Inputs=+++
  Discrete Transfer Fcn : DiscreteTransferFcn  Numerator=[1 -cos(w*Ts) 0]  Denominator=[1 -2*cos(w*Ts) 1]
  Discrete-Time Integrator : DiscreteIntegrator  gainval=1  SampleTime=-1  ICPrevOutput=DiscIntNeverNeededParam  ICPrevScaledInput=DiscIntNeverNeededParam
  Gain1 : Gain  Gain=Kp_U
  Gain2 : Gain  Gain=Kr_U
  Gain3 : Gain  Gain=Ki_U
  O : Outport
  wires:
  Gain1/1 -> Add/1
  I/1 -> Gain2/1, Gain3/1, Gain1/1
  Add/1 -> O/1
  Gain3/1 -> Discrete-Time Integrator/1
  Discrete-Time Integrator/1 -> Add/2
  Gain2/1 -> Discrete Transfer Fcn/1
  Discrete Transfer Fcn/1 -> Add/3

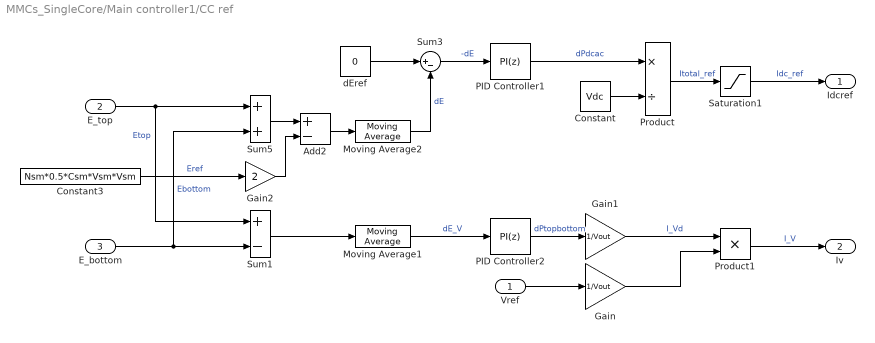
== system MMCs_SingleCore/Main controller1/CC ref ==
  Vref : Inport
  E_top : Inport  Port=2
  E_bottom : Inport  Port=3
  Add2 : Sum  Inputs=+-
  Constant : Constant  Value=Vdc
  Constant3 : Constant  Value=Nsm*0.5*Csm*Vsm*Vsm
  Gain : Gain  Gain=1/Vout
  Gain1 : Gain  Gain=1/Vout
  Gain2 : Gain  Gain=2
  Moving Average1 : eeGeneralControl/Moving Average  VariantControl=Variant1  LabelModeActiveChoice=Discrete  f=5  x0=0  BufferSize=8192  Ts=Ts
      settings: SourceProductBaseCode=PS
  Moving Average2 : eeGeneralControl/Moving Average  VariantControl=Variant1  LabelModeActiveChoice=Discrete  f=5  x0=0  BufferSize=8192  Ts=Ts
      settings: SourceProductBaseCode=PS
  PID Controller1 : slpidlib/PID Controller  Controller=PI  Form=Parallel  TimeDomain=Discrete-time  UseExternalTs=off  SampleTime=-1  IntegratorMethod=Forward Euler  FilterMethod=Forward Euler  ControllerParametersSource=internal  P=Kp_E1  I=Ki_E1  D=0  UseFilter=on  N=100  TunerSelectOption=Transfer Function Based (PID Tuner App)  InitialConditionSource=internal  InitialConditionForIntegrator=0  InitialConditionForFilter=0  DifferentiatorICPrevScaledInput=0  ExternalReset=none  TrackingMode=off  Kt=1  LimitOutput=off  SatLimitsSource=internal  UpperSaturationLimit=inf  LowerSaturationLimit=-inf  LinearizeAsGain=on  AntiWindupMode=none  Kb=1  POutMin=[]  POutMax=[]  IOutMin=[]  IOutMax=[]  DOutMin=[]  DOutMax=[]  NOutMin=[]  NOutMax=[]  SumOutMin=[]  SumOutMax=[]  SaturationOutMin=[]  SaturationOutMax=[]  PParamMin=[]  PParamMax=[]  IParamMin=[]  IParamMax=[]  DParamMin=[]  DParamMax=[]  NParamMin=[]  NParamMax=[]  KbParamMin=[]  KbParamMax=[]  KtParamMin=[]  KtParamMax=[]  KbOutMin=[]  KbOutMax=[]  KtOutMin=[]  KtOutMax=[]  IntegratorOutMin=[]  IntegratorOutMax=[]  FilterOutMin=[]  FilterOutMax=[]  SumI1OutMin=[]  SumI1OutMax=[]  SumI2OutMin=[]  SumI2OutMax=[]  SumI3OutMin=[]  SumI3OutMax=[]  SumI4OutMin=[]  SumI4OutMax=[]  SumDOutMin=[]  SumDOutMax=[]  DifferentiatorOutMin=[]  DifferentiatorOutMax=[]  FilterDiffOutCoefMin=[]  FilterDiffOutCoefMax=[]  ReciprocalOutMin=[]  ReciprocalOutMax=[]  SumDenOutMin=[]  SumDenOutMax=[]  SumNumOutMin=[]  SumNumOutMax=[]  DivideOutMin=[]  DivideOutMax=[]  UdiffTsProdOutMin=[]  UdiffTsProdOutMax=[]  NTsProdOutMin=[]  NTsProdOutMax=[]  UintegralTsProdOutMin=[]  UintegralTsProdOutMax=[]  UngainTsProdOutMin=[]  UngainTsProdOutMax=[]  IntegratorContinuousStateAttributes=''  IntegratorStateMustResolveToSignalObject=off  IntegratorRTWStateStorageClass=Auto  FilterContinuousStateAttributes=''  FilterStateMustResolveToSignalObject=off  FilterRTWStateStorageClass=Auto  ParallelPVariant=InternalParameters  IdealPVariant=Disabled  IVariant=InternalParameters  DVariant=Disabled  IntegratorVariant=Discrete  SatVariant=Disabled  AWVariant=Passthrough  PCopyVariant=Disabled  TRVariant=Disabled  FdbkBlocksVariant=Forward  IdealPFdbkVariant=Disabled  SatFdbkVariant=Disabled  DerivativeFilterVariant=Disabled  NVariant=Disabled  NCopyVariant=Disabled_SignalSpec  FilterICVariant=Disabled  IntegratorICVariant=InternalICs  ExternalResetVariant=Disabled  TRSumVariant=Passthrough  SumFdbkVariant=Disabled  SumVariant=Sum_PI  TsampFilterVariant=InternalTs  TsampNgainVariant=Passthrough  TsampIntegralVariant=Passthrough  ExternalSaturationOutDataTypeStr=Inherit: Same as second input
  PID Controller2 : slpidlib/PID Controller  Controller=PI  Form=Parallel  TimeDomain=Discrete-time  UseExternalTs=off  SampleTime=-1  IntegratorMethod=Forward Euler  FilterMethod=Forward Euler  ControllerParametersSource=internal  P=Kp_E2  I=Ki_E2  D=0  UseFilter=on  N=100  TunerSelectOption=Transfer Function Based (PID Tuner App)  InitialConditionSource=internal  InitialConditionForIntegrator=0  InitialConditionForFilter=0  DifferentiatorICPrevScaledInput=0  ExternalReset=none  TrackingMode=off  Kt=1  LimitOutput=off  SatLimitsSource=internal  UpperSaturationLimit=inf  LowerSaturationLimit=-inf  LinearizeAsGain=on  AntiWindupMode=none  Kb=1  POutMin=[]  POutMax=[]  IOutMin=[]  IOutMax=[]  DOutMin=[]  DOutMax=[]  NOutMin=[]  NOutMax=[]  SumOutMin=[]  SumOutMax=[]  SaturationOutMin=[]  SaturationOutMax=[]  PParamMin=[]  PParamMax=[]  IParamMin=[]  IParamMax=[]  DParamMin=[]  DParamMax=[]  NParamMin=[]  NParamMax=[]  KbParamMin=[]  KbParamMax=[]  KtParamMin=[]  KtParamMax=[]  KbOutMin=[]  KbOutMax=[]  KtOutMin=[]  KtOutMax=[]  IntegratorOutMin=[]  IntegratorOutMax=[]  FilterOutMin=[]  FilterOutMax=[]  SumI1OutMin=[]  SumI1OutMax=[]  SumI2OutMin=[]  SumI2OutMax=[]  SumI3OutMin=[]  SumI3OutMax=[]  SumI4OutMin=[]  SumI4OutMax=[]  SumDOutMin=[]  SumDOutMax=[]  DifferentiatorOutMin=[]  DifferentiatorOutMax=[]  FilterDiffOutCoefMin=[]  FilterDiffOutCoefMax=[]  ReciprocalOutMin=[]  ReciprocalOutMax=[]  SumDenOutMin=[]  SumDenOutMax=[]  SumNumOutMin=[]  SumNumOutMax=[]  DivideOutMin=[]  DivideOutMax=[]  UdiffTsProdOutMin=[]  UdiffTsProdOutMax=[]  NTsProdOutMin=[]  NTsProdOutMax=[]  UintegralTsProdOutMin=[]  UintegralTsProdOutMax=[]  UngainTsProdOutMin=[]  UngainTsProdOutMax=[]  IntegratorContinuousStateAttributes=''  IntegratorStateMustResolveToSignalObject=off  IntegratorRTWStateStorageClass=Auto  FilterContinuousStateAttributes=''  FilterStateMustResolveToSignalObject=off  FilterRTWStateStorageClass=Auto  ParallelPVariant=InternalParameters  IdealPVariant=Disabled  IVariant=InternalParameters  DVariant=Disabled  IntegratorVariant=Discrete  SatVariant=Disabled  AWVariant=Passthrough  PCopyVariant=Disabled  TRVariant=Disabled  FdbkBlocksVariant=Forward  IdealPFdbkVariant=Disabled  SatFdbkVariant=Disabled  DerivativeFilterVariant=Disabled  NVariant=Disabled  NCopyVariant=Disabled_SignalSpec  FilterICVariant=Disabled  IntegratorICVariant=InternalICs  ExternalResetVariant=Disabled  TRSumVariant=Passthrough  SumFdbkVariant=Disabled  SumVariant=Sum_PI  TsampFilterVariant=InternalTs  TsampNgainVariant=Passthrough  TsampIntegralVariant=Passthrough  ExternalSaturationOutDataTypeStr=Inherit: Same as second input
  Product : Product  Inputs=*/  InputSameDT=on  SaturateOnIntegerOverflow=on  OutDataTypeStr=Inherit: Same as first input
  Product1 : Product
  Saturation1 : Saturate  UpperLimit=1  LowerLimit=-1
  Sum1 : Sum  Inputs=+-
  Sum3 : Sum  Inputs=|+-
  Sum5 : Sum
  dEref : Constant  Value=0
  Idcref : Outport
  Iv : Outport  Port=2
  wires:
  Add2/1 -> Moving Average2/1
  Gain2/1 -> Add2/2
  Constant3/1 -> Gain2/1  "Eref"
  Gain1/1 -> Product1/1  "I_Vd"
  Product/1 -> Saturation1/1  "Itotal_ref"
  Gain/1 -> Product1/2
  Product1/1 -> Iv/1  "I_V"
  E_bottom/1 -> Sum1/2, Sum5/2  "Ebottom"
  E_top/1 -> Sum1/1, Sum5/1  "Etop"
  Saturation1/1 -> Idcref/1  "Idc_ref"
  PID Controller2/1 -> Gain1/1  "dPtopbottom"
  Moving Average1/1 -> PID Controller2/1  "dE_V"
  Sum1/1 -> Moving Average1/1
  PID Controller1/1 -> Product/1  "dPdcac"
  Sum3/1 -> PID Controller1/1  "-dE"
  dEref/1 -> Sum3/1
  Moving Average2/1 -> Sum3/2  "dE"
  Sum5/1 -> Add2/1
  Constant/1 -> Product/2
  Vref/1 -> Gain/1

== system MMCs_SingleCore/Main controller1/PR 1 ==
  I : Inport
  Add : Sum  Inputs=+++
  Discrete Transfer Fcn : DiscreteTransferFcn  Numerator=[1 -cos(w*Ts) 0]  Denominator=[1 -2*cos(w*Ts) 1]
  Discrete-Time Integrator : DiscreteIntegrator  gainval=1  SampleTime=-1  ICPrevOutput=DiscIntNeverNeededParam  ICPrevScaledInput=DiscIntNeverNeededParam
  Gain1 : Gain  Gain=Kp_I
  Gain2 : Gain  Gain=Kr_I
  Gain3 : Gain  Gain=Ki_I
  O : Outport
  wires:
  Discrete-Time Integrator/1 -> Add/2
  Gain3/1 -> Discrete-Time Integrator/1
  Discrete Transfer Fcn/1 -> Add/3
  Gain2/1 -> Discrete Transfer Fcn/1
  Gain1/1 -> Add/1
  I/1 -> Gain1/1, Gain3/1, Gain2/1
  Add/1 -> O/1

== system MMCs_SingleCore/Main controller1/PR 2 ==
  I : Inport
  Add : Sum  Inputs=+++
  Discrete Transfer Fcn : DiscreteTransferFcn  Numerator=[1 -cos(w*Ts) 0]  Denominator=[1 -2*cos(w*Ts) 1]
  Discrete-Time Integrator : DiscreteIntegrator  gainval=1  SampleTime=-1  ICPrevOutput=DiscIntNeverNeededParam  ICPrevScaledInput=DiscIntNeverNeededParam
  Gain1 : Gain  Gain=Kp_cc
  Gain2 : Gain  Gain=Kr_cc
  Gain3 : Gain  Gain=Ki_cc
  O : Outport
  wires:
  Discrete-Time Integrator/1 -> Add/2  "I"
  Gain3/1 -> Discrete-Time Integrator/1
  Add/1 -> O/1
  Discrete Transfer Fcn/1 -> Add/3  "R"
  I/1 -> Gain1/1, Gain3/1, Gain2/1  "In"
  Gain1/1 -> Add/1  "P"
  Gain2/1 -> Discrete Transfer Fcn/1

== system MMCs_SingleCore/Main controller1/PR Controller ==
  I : Inport
  Add : Sum  Inputs=+++
  Discrete Transfer Fcn : DiscreteTransferFcn  Numerator=[1 -cos(w*Ts) 0]  Denominator=[1 -2*cos(w*Ts) 1]
  Discrete-Time Integrator : DiscreteIntegrator  gainval=1  SampleTime=-1  ICPrevOutput=DiscIntNeverNeededParam  ICPrevScaledInput=DiscIntNeverNeededParam
  Gain1 : Gain  Gain=Kp_U
  Gain2 : Gain  Gain=Kr_U
  Gain3 : Gain  Gain=Ki_U
  O : Outport
  wires:
  Discrete Transfer Fcn/1 -> Add/3
  Gain2/1 -> Discrete Transfer Fcn/1
  Discrete-Time Integrator/1 -> Add/2
  Gain3/1 -> Discrete-Time Integrator/1
  Add/1 -> O/1
  I/1 -> Gain1/1, Gain3/1, Gain2/1
  Gain1/1 -> Add/1

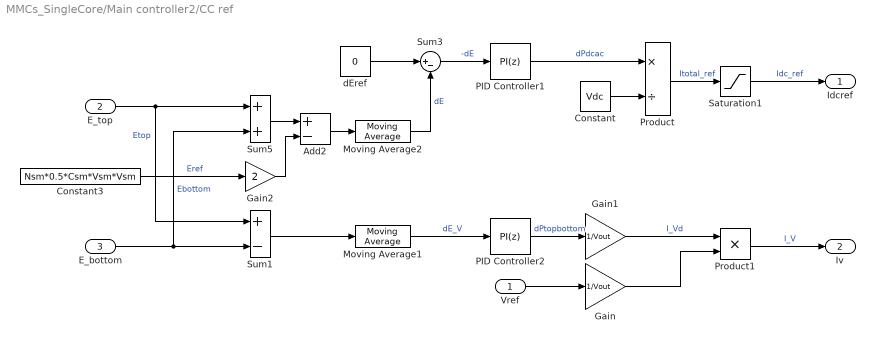
== system MMCs_SingleCore/Main controller2/CC ref ==
  Vref : Inport
  E_top : Inport  Port=2
  E_bottom : Inport  Port=3
  Add2 : Sum  Inputs=+-
  Constant : Constant  Value=Vdc
  Constant3 : Constant  Value=Nsm*0.5*Csm*Vsm*Vsm
  Gain : Gain  Gain=1/Vout
  Gain1 : Gain  Gain=1/Vout
  Gain2 : Gain  Gain=2
  Moving Average1 : eeGeneralControl/Moving Average  VariantControl=Variant1  LabelModeActiveChoice=Discrete  f=5  x0=0  BufferSize=8192  Ts=Ts
      settings: SourceProductBaseCode=PS
  Moving Average2 : eeGeneralControl/Moving Average  VariantControl=Variant1  LabelModeActiveChoice=Discrete  f=5  x0=0  BufferSize=8192  Ts=Ts
      settings: SourceProductBaseCode=PS
  PID Controller1 : slpidlib/PID Controller  Controller=PI  Form=Parallel  TimeDomain=Discrete-time  UseExternalTs=off  SampleTime=-1  IntegratorMethod=Forward Euler  FilterMethod=Forward Euler  ControllerParametersSource=internal  P=Kp_E1  I=Ki_E1  D=0  UseFilter=on  N=100  TunerSelectOption=Transfer Function Based (PID Tuner App)  InitialConditionSource=internal  InitialConditionForIntegrator=0  InitialConditionForFilter=0  DifferentiatorICPrevScaledInput=0  ExternalReset=none  TrackingMode=off  Kt=1  LimitOutput=off  SatLimitsSource=internal  UpperSaturationLimit=inf  LowerSaturationLimit=-inf  LinearizeAsGain=on  AntiWindupMode=none  Kb=1  POutMin=[]  POutMax=[]  IOutMin=[]  IOutMax=[]  DOutMin=[]  DOutMax=[]  NOutMin=[]  NOutMax=[]  SumOutMin=[]  SumOutMax=[]  SaturationOutMin=[]  SaturationOutMax=[]  PParamMin=[]  PParamMax=[]  IParamMin=[]  IParamMax=[]  DParamMin=[]  DParamMax=[]  NParamMin=[]  NParamMax=[]  KbParamMin=[]  KbParamMax=[]  KtParamMin=[]  KtParamMax=[]  KbOutMin=[]  KbOutMax=[]  KtOutMin=[]  KtOutMax=[]  IntegratorOutMin=[]  IntegratorOutMax=[]  FilterOutMin=[]  FilterOutMax=[]  SumI1OutMin=[]  SumI1OutMax=[]  SumI2OutMin=[]  SumI2OutMax=[]  SumI3OutMin=[]  SumI3OutMax=[]  SumI4OutMin=[]  SumI4OutMax=[]  SumDOutMin=[]  SumDOutMax=[]  DifferentiatorOutMin=[]  DifferentiatorOutMax=[]  FilterDiffOutCoefMin=[]  FilterDiffOutCoefMax=[]  ReciprocalOutMin=[]  ReciprocalOutMax=[]  SumDenOutMin=[]  SumDenOutMax=[]  SumNumOutMin=[]  SumNumOutMax=[]  DivideOutMin=[]  DivideOutMax=[]  UdiffTsProdOutMin=[]  UdiffTsProdOutMax=[]  NTsProdOutMin=[]  NTsProdOutMax=[]  UintegralTsProdOutMin=[]  UintegralTsProdOutMax=[]  UngainTsProdOutMin=[]  UngainTsProdOutMax=[]  IntegratorContinuousStateAttributes=''  IntegratorStateMustResolveToSignalObject=off  IntegratorRTWStateStorageClass=Auto  FilterContinuousStateAttributes=''  FilterStateMustResolveToSignalObject=off  FilterRTWStateStorageClass=Auto  ParallelPVariant=InternalParameters  IdealPVariant=Disabled  IVariant=InternalParameters  DVariant=Disabled  IntegratorVariant=Discrete  SatVariant=Disabled  AWVariant=Passthrough  PCopyVariant=Disabled  TRVariant=Disabled  FdbkBlocksVariant=Forward  IdealPFdbkVariant=Disabled  SatFdbkVariant=Disabled  DerivativeFilterVariant=Disabled  NVariant=Disabled  NCopyVariant=Disabled_SignalSpec  FilterICVariant=Disabled  IntegratorICVariant=InternalICs  ExternalResetVariant=Disabled  TRSumVariant=Passthrough  SumFdbkVariant=Disabled  SumVariant=Sum_PI  TsampFilterVariant=InternalTs  TsampNgainVariant=Passthrough  TsampIntegralVariant=Passthrough  ExternalSaturationOutDataTypeStr=Inherit: Same as second input
  PID Controller2 : slpidlib/PID Controller  Controller=PI  Form=Parallel  TimeDomain=Discrete-time  UseExternalTs=off  SampleTime=-1  IntegratorMethod=Forward Euler  FilterMethod=Forward Euler  ControllerParametersSource=internal  P=Kp_E2  I=Ki_E2  D=0  UseFilter=on  N=100  TunerSelectOption=Transfer Function Based (PID Tuner App)  InitialConditionSource=internal  InitialConditionForIntegrator=0  InitialConditionForFilter=0  DifferentiatorICPrevScaledInput=0  ExternalReset=none  TrackingMode=off  Kt=1  LimitOutput=off  SatLimitsSource=internal  UpperSaturationLimit=inf  LowerSaturationLimit=-inf  LinearizeAsGain=on  AntiWindupMode=none  Kb=1  POutMin=[]  POutMax=[]  IOutMin=[]  IOutMax=[]  DOutMin=[]  DOutMax=[]  NOutMin=[]  NOutMax=[]  SumOutMin=[]  SumOutMax=[]  SaturationOutMin=[]  SaturationOutMax=[]  PParamMin=[]  PParamMax=[]  IParamMin=[]  IParamMax=[]  DParamMin=[]  DParamMax=[]  NParamMin=[]  NParamMax=[]  KbParamMin=[]  KbParamMax=[]  KtParamMin=[]  KtParamMax=[]  KbOutMin=[]  KbOutMax=[]  KtOutMin=[]  KtOutMax=[]  IntegratorOutMin=[]  IntegratorOutMax=[]  FilterOutMin=[]  FilterOutMax=[]  SumI1OutMin=[]  SumI1OutMax=[]  SumI2OutMin=[]  SumI2OutMax=[]  SumI3OutMin=[]  SumI3OutMax=[]  SumI4OutMin=[]  SumI4OutMax=[]  SumDOutMin=[]  SumDOutMax=[]  DifferentiatorOutMin=[]  DifferentiatorOutMax=[]  FilterDiffOutCoefMin=[]  FilterDiffOutCoefMax=[]  ReciprocalOutMin=[]  ReciprocalOutMax=[]  SumDenOutMin=[]  SumDenOutMax=[]  SumNumOutMin=[]  SumNumOutMax=[]  DivideOutMin=[]  DivideOutMax=[]  UdiffTsProdOutMin=[]  UdiffTsProdOutMax=[]  NTsProdOutMin=[]  NTsProdOutMax=[]  UintegralTsProdOutMin=[]  UintegralTsProdOutMax=[]  UngainTsProdOutMin=[]  UngainTsProdOutMax=[]  IntegratorContinuousStateAttributes=''  IntegratorStateMustResolveToSignalObject=off  IntegratorRTWStateStorageClass=Auto  FilterContinuousStateAttributes=''  FilterStateMustResolveToSignalObject=off  FilterRTWStateStorageClass=Auto  ParallelPVariant=InternalParameters  IdealPVariant=Disabled  IVariant=InternalParameters  DVariant=Disabled  IntegratorVariant=Discrete  SatVariant=Disabled  AWVariant=Passthrough  PCopyVariant=Disabled  TRVariant=Disabled  FdbkBlocksVariant=Forward  IdealPFdbkVariant=Disabled  SatFdbkVariant=Disabled  DerivativeFilterVariant=Disabled  NVariant=Disabled  NCopyVariant=Disabled_SignalSpec  FilterICVariant=Disabled  IntegratorICVariant=InternalICs  ExternalResetVariant=Disabled  TRSumVariant=Passthrough  SumFdbkVariant=Disabled  SumVariant=Sum_PI  TsampFilterVariant=InternalTs  TsampNgainVariant=Passthrough  TsampIntegralVariant=Passthrough  ExternalSaturationOutDataTypeStr=Inherit: Same as second input
  Product : Product  Inputs=*/  InputSameDT=on  SaturateOnIntegerOverflow=on  OutDataTypeStr=Inherit: Same as first input
  Product1 : Product
  Saturation1 : Saturate  UpperLimit=1  LowerLimit=-1
  Sum1 : Sum  Inputs=+-
  Sum3 : Sum  Inputs=|+-
  Sum5 : Sum
  dEref : Constant  Value=0
  Idcref : Outport
  Iv : Outport  Port=2
  wires:
  Vref/1 -> Gain/1
  Constant/1 -> Product/2
  Sum5/1 -> Add2/1
  Moving Average2/1 -> Sum3/2  "dE"
  dEref/1 -> Sum3/1
  Sum3/1 -> PID Controller1/1  "-dE"
  PID Controller1/1 -> Product/1  "dPdcac"
  Sum1/1 -> Moving Average1/1
  Moving Average1/1 -> PID Controller2/1  "dE_V"
  PID Controller2/1 -> Gain1/1  "dPtopbottom"
  Saturation1/1 -> Idcref/1  "Idc_ref"
  E_top/1 -> Sum5/1, Sum1/1  "Etop"
  E_bottom/1 -> Sum5/2, Sum1/2  "Ebottom"
  Product1/1 -> Iv/1  "I_V"
  Gain/1 -> Product1/2
  Product/1 -> Saturation1/1  "Itotal_ref"
  Gain1/1 -> Product1/1  "I_Vd"
  Constant3/1 -> Gain2/1  "Eref"
  Gain2/1 -> Add2/2
  Add2/1 -> Moving Average2/1

== system MMCs_SingleCore/Main controller2/PR 1 ==
  I : Inport
  Add : Sum  Inputs=+++
  Discrete Transfer Fcn : DiscreteTransferFcn  Numerator=[1 -cos(w*Ts) 0]  Denominator=[1 -2*cos(w*Ts) 1]
  Discrete-Time Integrator : DiscreteIntegrator  gainval=1  SampleTime=-1  ICPrevOutput=DiscIntNeverNeededParam  ICPrevScaledInput=DiscIntNeverNeededParam
  Gain1 : Gain  Gain=Kp_I
  Gain2 : Gain  Gain=Kr_I
  Gain3 : Gain  Gain=Ki_I
  O : Outport
  wires:
  Add/1 -> O/1
  I/1 -> Gain2/1, Gain3/1, Gain1/1
  Gain1/1 -> Add/1
  Gain2/1 -> Discrete Transfer Fcn/1
  Discrete Transfer Fcn/1 -> Add/3
  Gain3/1 -> Discrete-Time Integrator/1
  Discrete-Time Integrator/1 -> Add/2

== system MMCs_SingleCore/Main controller2/PR 2 ==
  I : Inport
  Add : Sum  Inputs=+++
  Discrete Transfer Fcn : DiscreteTransferFcn  Numerator=[1 -cos(w*Ts) 0]  Denominator=[1 -2*cos(w*Ts) 1]
  Discrete-Time Integrator : DiscreteIntegrator  gainval=1  SampleTime=-1  ICPrevOutput=DiscIntNeverNeededParam  ICPrevScaledInput=DiscIntNeverNeededParam
  Gain1 : Gain  Gain=Kp_cc
  Gain2 : Gain  Gain=Kr_cc
  Gain3 : Gain  Gain=Ki_cc
  O : Outport
  wires:
  Gain2/1 -> Discrete Transfer Fcn/1
  Gain1/1 -> Add/1  "P"
  I/1 -> Gain2/1, Gain3/1, Gain1/1  "In"
  Discrete Transfer Fcn/1 -> Add/3  "R"
  Add/1 -> O/1
  Gain3/1 -> Discrete-Time Integrator/1
  Discrete-Time Integrator/1 -> Add/2  "I"

== system MMCs_SingleCore/Main controller2/PR Controller ==
  I : Inport
  Add : Sum  Inputs=+++
  Discrete Transfer Fcn : DiscreteTransferFcn  Numerator=[1 -cos(w*Ts) 0]  Denominator=[1 -2*cos(w*Ts) 1]
  Discrete-Time Integrator : DiscreteIntegrator  gainval=1  SampleTime=-1  ICPrevOutput=DiscIntNeverNeededParam  ICPrevScaledInput=DiscIntNeverNeededParam
  Gain1 : Gain  Gain=Kp_U
  Gain2 : Gain  Gain=Kr_U
  Gain3 : Gain  Gain=Ki_U
  O : Outport
  wires:
  Gain1/1 -> Add/1
  I/1 -> Gain2/1, Gain3/1, Gain1/1
  Add/1 -> O/1
  Gain3/1 -> Discrete-Time Integrator/1
  Discrete-Time Integrator/1 -> Add/2
  Gain2/1 -> Discrete Transfer Fcn/1
  Discrete Transfer Fcn/1 -> Add/3
